simulink model "PID_Loop_2024a"  (R2024b)
settings: Solver=FixedStepAuto  StartTime=0.0  StopTime=tspan  FixedStep=dt  RelTol=1e-3
model workspace (MAT data in the model file):
  Drag_Constants = 1
  mass = [5.51 5.51 5.51 1 1 1]
  mass_6a = [5 5 5 1 1 1]
values from neighbouring files (symbols this model uses):
  acc_bias_instability = 19e-6*9.81    (= 0.00018639)    [init.m]
  acc_noise = 60e-6*9.81    (= 0.0005886)    [init.m]
  acc_vel_rw = 0.02/sqrt(3600)    [init.m]
  do_bouyancy_flag = 1    [PID_testing_data_producer.m]    (also in init.m = 0)
  do_gravity_flag = 1    [PID_testing_data_producer.m]    (also in init.m = 0)
  do_imu_noise_flag = 0    [PID_testing_data_producer.m]    (also in init.m)
  dt = 0.001    [PID_testing_data_producer.m]    (also in init.m)
  Dt = 0.01    [init.m]
  g = 9.8067    [constants.m]    (also in constants.mat = 9.80665)
  gyro_bias_instability = 1.5/3600/360    (= 1.15740740741e-06)    [init.m]
  gyro_noise = 5e-3*2*pi/360    (= 8.72664625997e-05)    [init.m]
  gyro_rw = 0.16*2*pi/360/sqrt(3600)    [init.m]
  H = [1 0 0 ... (first row only)    [init.m]
  inverse_wrench = pinv(wrench)    [calculate_wrench.m]    (also in constants.m = geometry_properties.inverse_wrench; geometry_properties.mat = [0.09 0.09 -0.09 -0.09 0.353553390593 0.353553390593 0.35355)
  mag_noise = 0.1    [init.m]
  max_pitch_torque = norm(wrench*(F_max*[1 1 -1 -1 0 0 0 0]'))    [calculate_wrench.m]
  max_roll_torque = norm(wrench*(F_max*[1 -1 1 -1 0 0 0 0]'))    [calculate_wrench.m]
  max_yaw_torque = norm(wrench*(F_max*[0 0 0 0 -1 1 -1 1]'))    [calculate_wrench.m]
  pitch_force = [0         0         0         0    1.0000         0]    [constants.m]
  plot_dt = 0.01    [init.m]
  Q = diag([0.0001, 0.0001, 0.1])    [init.m]
  R = [.1 0 ... (first row only)    [init.m]
  roll_force = [0         0         0    0.5000         0         0]    [constants.m]
  states_desired = [x_des;E_des]    [init.m]
  volume = 0.0074    [constants.m]    (also in constants.mat = 0.0073741788)
  volume_center = [0, 0, 0.1]    [constants.m]    (also in constants.mat = [0 0 0.1])
  water_density = 997    [constants.m]    (also in constants.mat = 1000)
  waypoints = input_state_errors(:,i)    [PID_testing_data_producer.m]    (also in init.m = [0, 0, 0])
  wrench = eval(w)    [calculate_wrench.m]    (also in constants.m = geometry_properties.wrench; constants.mat = [0 0 0 0 -0.7071 -0.7071 -0.7071 -0.7071 0 0 0 0 ... (48 ele; geometry_properties.mat = [0 0 -1 0.22 0.25 0 0 0 -1 -0.22 0.25 0 ... (48 elements, 6x; wrench.m)
  x_force = [0.4100         0         0         0         0         0]    [constants.m]    (also in init2.m = [0.410000000000000	0	0	0	0	0])
  y_force = [0    0.5000         0         0         0         0]    [constants.m]    (also in init2.m = [0	0.500000000000000	0	0	0	0])
  yaw_force = [0         0         0         0         0    0.5000]    [constants.m]
  z_force = [0         0    1.2500         0         0         0]    [constants.m]
undefined symbols (not defined in the file or in its folder): E0_est, fractalcoef, IMU, P, v0_e_est, x0_e_est
libraries: slpidlib x4, mspsensorlib x2, shared6dof x1, simulink x1, sharedTrackingLibrary x1, uavutilslib x1
(part 2 of 2)

== matlab function PID_Loop_2024a/Plant/Thruster Forces/PWM to Motor Forces ==
  data: thruster_pwms input; forces_N output; P input
function forces_N  = fcn(thruster_pwms, P)
    %{
        This function  uses a polynomial fit to the pwm vs thrust curve 
        for the T200 Thrusters to calculate the 8 thruster force vectors.
    %}
    %preallocate
    forces_N = zeros(size(thruster_pwms)); 
    
    
    % First condition: 1100 <= x < 1460
    index_array = (thruster_pwms >= 1100 & thruster_pwms < 1460);

    
    forces_N(index_array) =  (-1.76709811615214e-07) * thruster_pwms(index_array).^3 ...
                 + (0.000566300482093069) * thruster_pwms(index_array).^2 ...
                 + (-0.478920592563405) * thruster_pwms(index_array) ...
                 + 41.55273858905;
    
    % Second condition: 1460 <= x <= 1540
    index_array = (thruster_pwms >= 1460 & thruster_pwms <= 1540);
    forces_N(index_array) = 0;
    
    % Third condition: 1540 < x <= 1900
    index_array = (thruster_pwms > 1540 & thruster_pwms <= 1900);
    forces_N(index_array) = (-1.81933850672702e-07) * thruster_pwms(index_array).^3 ...
                 + (0.00109777888824906) * thruster_pwms(index_array).^2 ...
                 + (-2.03121269418349) * thruster_pwms(index_array) ...
                 + (1189.65910925401);
    
    % Handle out-of-range values
    if any(isnan(forces_N))
        error('Some values in x_array are out of the valid range [1100..1900].');
    end

    
end

== matlab function PID_Loop_2024a/SPU/Temporary Brute Force Integration/Inverted Attitude Kinematics ==
  data: w_est input; dE_est output; E_est input
function dE_est = fcn(w_est,E_est)
%unpack Euler angles
phi = E_est(1);
theta = E_est(2);
psi = E_est(3);

dE_est = [1, sin(phi)*tan(theta), cos(phi)*tan(theta);...
    0, cos(phi), -sin(phi);...
    0, sin(phi)/cos(theta), cos(phi)/cos(theta)]*w_est;

== matlab function PID_Loop_2024a/Controller/Thruster Forces to PWM ==
  data: thruster_force_cmd input; pwm_cmd output
function pwm_cmd = fcn(thruster_force_cmd)

pwm_cmd = zeros(8,1);
%uses a curve fit for thrust to pwm from the t200 thruster data sheet

for i=1:length(pwm_cmd)
    x = thruster_force_cmd(i);
    y = 0;

    if(x>0)
        y = round(0.00231011300235566*x^3 + -0.229204832763592*x^2 + 13.7272237851422*x + 1536.34500151024);
    elseif(x<0)
        y = round(0.00475737746846442*x^3 + 0.360062809963915*x^2 + 17.2034080439155*x + 1463.91061014397);
    else
        y = 1500;
    end

    %saturation
    if(y > 1900)
        y = 1900;
    end
    if (y < 1100)
        y = 1100;
    end

    pwm_cmd(i) = y;

end

== matlab function PID_Loop_2024a/Plant/Static Forces and Torques/Bouyant Force ==
  data: DCMbe input; buoyant_force output; g parameter; water_density parameter; volume parameter; volume_center parameter
function buoyant_force = buoyant_force(DCMbe, g, water_density, volume, volume_center)

    % Ensure d is a column vector
    volume_center = volume_center(:);

    % Buoyant force vector in world frame
    b_vector = [0; 0; water_density * -g * volume];

    % Rotate buoyant force to object's frame
    buoyant_force_body = DCMbe * b_vector;

    % Compute torque using cross product τ = d × F_buoyancy
    % (MATLAB cross function works for column vectors)
    torque = cross(-volume_center, buoyant_force_body);

    % Combine force and torque into a single output vector
    buoyant_force = [buoyant_force_body; torque];
end

== matlab function PID_Loop_2024a/Plant/Static Forces and Torques/Weight ==
  data: DCMbe input; weight_force output; g parameter; P parameter
function weight_force = weight_force(DCMbe, g, P)
    m = P.m;

    % Gravity force vector in world frame (downward)
    g_vector = [0; 0; m * g];
    
    % Linear Force
    lin = DCMbe * g_vector;
    % Rotational force
    rot = [0;0;0];
    % Transform gravity force to rotated frame
    weight_force = [lin; rot];
end

== matlab function PID_Loop_2024a/Waypoint Follower/Desired State Generator ==
  data: current_waypoint output; waypoints input; desired_states output; states_des input; current_waypoint_index output; current_waypoint_index input; intermediate_waypoint input; tol parameter; intermediate_waypoint output
function [current_waypoint,desired_states,current_waypoint_index,intermediate_waypoint]= fcn(waypoints,states_des,current_waypoint_index,intermediate_waypoint,tol)

%The initial value of the current_waypoint_index is 1, as set in the data
%store memory block.
x_e = states_des(1:3);

% check the next waypoint in the list
current_waypoint = waypoints(:,current_waypoint_index);

%get the length of the waypoint list
[~, N_wp] = size(waypoints);
% get the position vector to the current waypoint
r_b2wp_e = current_waypoint - x_e;
%get the range to the current waypoint
R_wp = norm(r_b2wp_e);

% get the range to the current intermediate waypoint
r_b2iwp_e = intermediate_waypoint - x_e;
R_int_wp = norm(r_b2iwp_e);

% if the range to the intermediate waypoint is smaller than the tolerance
if(R_wp <= tol)
    %if there is another waypoint on the list, switch the current waypoint
    %to that
    if(current_waypoint_index < N_wp)
        current_waypoint_index = current_waypoint_index + 1; %update wp index
        current_waypoint = waypoints(:,current_waypoint_index); %update wp
    else
        %keep using the current waypoint without changing it
        current_waypoint_index = N_wp;
        current_waypoint = current_waypoint; 
    end
    %recalculate the range
    r_b2wp_e = current_waypoint - x_e;
    R_wp = norm(r_b2wp_e);
end

%if the range to the waypoint and intermediate waypoint is larger than 1
if(R_wp > 1 && R_int_wp > 1)
    %create an intermediate waypoint
    intermediate_waypoint = x_e + r_b2wp_e/R_wp;
    r_b2iwp_e = intermediate_waypoint - x_e;
    R_int_wp = norm(r_b2iwp_e);

%if the range to the waypoint is greater than 1 but the vehicle is close
%the intermediate waypoint 
elseif(R_wp > 1 && R_int_wp <= 1 && R_int_wp > tol)
    %keep using the intermediate waypoint
    intermediate_waypoint = intermediate_waypoint;

%if the vehicle is far from the current waypoint but has reached the
%intermediate waypoint
elseif(R_wp > 1 && R_int_wp <= tol)
    %generate a new intermediate waypoint
    intermediate_waypoint = x_e + r_b2wp_e/R_wp;

%if the vehicle is close to the final waypoint, make the intermediate
%waypoint the final waypoint
elseif(R_wp <= 1)
    intermediate_waypoint = current_waypoint;

else
    %this shouldn't be reached, but here just in case
    intermediate_waypoint = current_waypoint;
end

%bearing angle
E = states_des(4:6); %unpack the euler angles
DCMbe = eul2rotm(E'); %calculate the rotation matrix
r_b2iwp_b = DCMbe*r_b2iwp_e; %calculate the bearing vector in the body frame
%xy_r_b2iwp_b = [r_b2iwp_b(1); r_b2iwp_b(2); 0]; %project onto xy plane

%to do: figure this out
yaw = atan2(r_b2iwp_b(1),r_b2iwp_b(2));

%put on interval -pi to pi
if (yaw > pi)
    yaw = yaw - 2*pi;
end

desired_states = [intermediate_waypoint;[0 0 yaw]'];

end

== matlab function PID_Loop_2024a/Attitude EKF/Euler EKF ==
  data: phi_meas input; theta_meas input; phi_hat output; w_meas input; xhat_prior input; P_prior input; theta_hat output; psi_hat output; dt parameter; H parameter; x output; P output; Q parameter; R parameter
function [phi_hat, theta_hat, psi_hat, x, P] = fcn(phi_meas,theta_meas,w_meas,xhat_prior,P_prior,dt, H, Q, R)

%Inputs: 
%   z = [phi_meas, theta_meas]', the measured euler angles
%   w = [p q r]' the measured angular rates
%   dt = timestep

%changed variable names to match source material
z = [phi_meas, theta_meas]';
x = xhat_prior;
rates = w_meas;
P = P_prior;

A = Ajacob(x, rates, dt); %get state transition matrix from linearization

%Predict
xp = fx(x, rates, dt); %use state transition function to get a priori update of states
Pp = A*P*A' + Q; %compute a priori error covariance matrix

K = Pp*H'*inv(H*Pp*H' + R); %compute kalman gain

%Correct using measurements
x = xp + K*(z - H*xp);
P = Pp - K*H*Pp;

%use built in matlab functions to make sure euler angles are in the correct
%domain
eul = [x(1) x(2) x(3)];
rotmZXY = eul2rotm(eul);
eul = rotm2eul(rotmZXY);

%outputs
phi_hat = eul(1);
theta_hat = eul(2);
psi_hat = eul(3);
x = [phi_hat;theta_hat;psi_hat];



%state transition function
function xp = fx(xhat,rates,dt)
    phi = xhat(1);
    theta = xhat(2);

    p = rates(1);
    q = rates(2);
    r = rates(3);

    xdot = zeros(3,1);

    %euler angle kinematics
    xdot(1) = p + q*sin(phi)*tan(theta) + r*cos(phi)*tan(theta);
    xdot(2) = q*cos(phi) - r*sin(phi);
    xdot(3) = q*sin(phi)*sec(theta) + r*cos(phi)*sec(theta);

    xp = xhat + xdot*dt;

end

%jacobian function
function A = Ajacob(xhat, rates, dt)
    A = zeros(3,3);

    phi = xhat(1);
    theta = xhat(2);

    p = rates(1);
    q = rates(2);
    r = rates(3);

    A(1,1) = q*cos(phi)*tan(theta) - r*sin(phi)*tan(theta);
    A(1,2) = q*sin(phi)*sec(theta)^2 - r*cos(phi)*sec(theta)^2;
    A(1,3) = 0;

    A(2,1) = -q*sin(phi) - r*cos(phi);
    A(2,2) = 0;
    A(2,3) = 0;

    A(3,1) = q*cos(phi)*sec(theta) - r*sin(phi)*sec(theta);
    A(3,2) = q*sin(phi)*sec(theta)*tan(theta) + r*cos(phi)*sec(theta)*tan(theta);
    A(3,3) = 0;

    A = eye(3) + A*dt;
end
end
